simulink model "StewartDynamics"  (R2015a)
settings: Solver=ode45  StartTime=0.0  StopTime=10.0  RelTol=1e-3
settings Model: Creator=admin  LastModifiedBy=admin

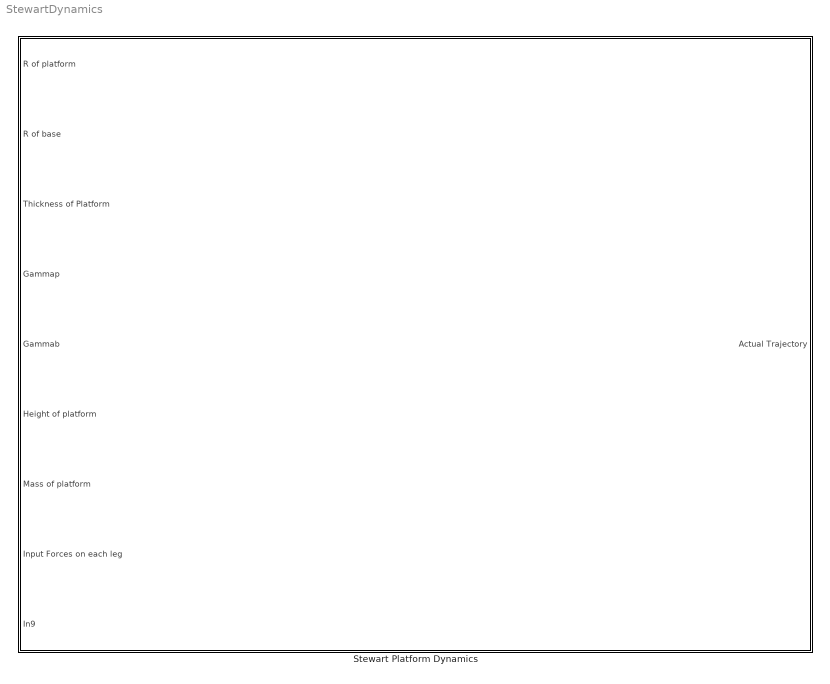
== system StewartDynamics ==
  Stewart Platform Dynamics : Subsystem

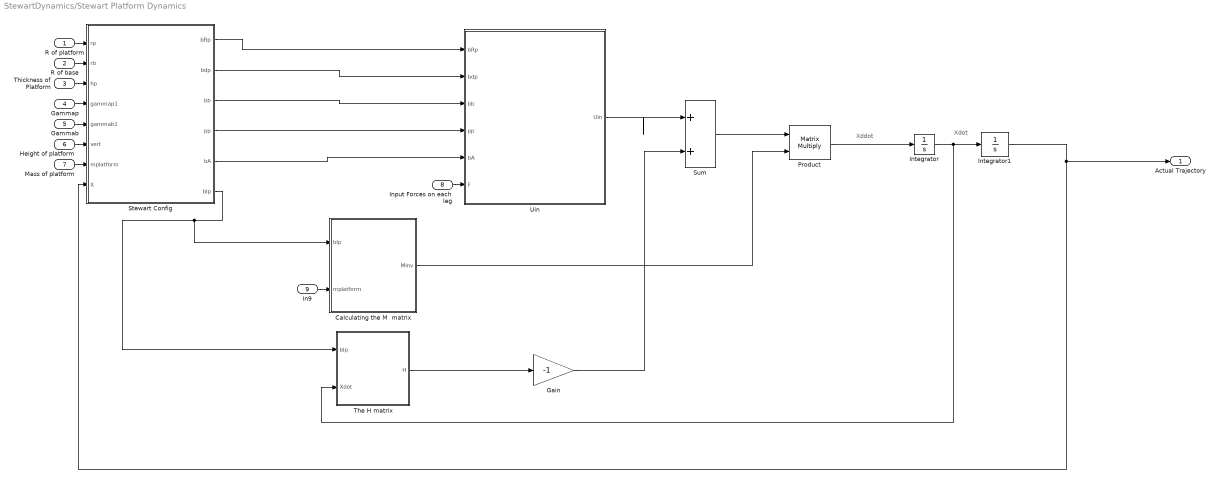
== system StewartDynamics/Stewart Platform Dynamics ==
  note: Xdot
  note: Xddot
  R of platform : Inport
  R of base : Inport  Port=2
  Thickness of Platform : Inport  Port=3
  Gammap : Inport  Port=4
  Gammab : Inport  Port=5
  "Height of platform " : Inport  Port=6
  Mass of platform : Inport  Port=7
  Input Forces on each leg : Inport  Port=8
  In9 : Inport  Port=9
  Calculating the M  matrix : MATLAB Function  TreatAsAtomicUnit=on
  Gain : Gain  Gain=-1
  Integrator : Integrator
  Integrator1 : Integrator
  Product : Product  Multiplication=Matrix(*)
  Stewart Config : MATLAB Function  TreatAsAtomicUnit=on
  Sum : Sum  Inputs=|++
  The H matrix : MATLAB Function  TreatAsAtomicUnit=on
  Uin : MATLAB Function  TreatAsAtomicUnit=on
  Actual Trajectory : Outport
  wires:
  R of platform/1 -> Stewart Config/1(rp)
  "Height of platform "/1 -> Stewart Config/6(vert)
  Input Forces on each leg/1 -> Uin/6(F)
  Gammap/1 -> Stewart Config/4(gammap1)
  Gammab/1 -> Stewart Config/5(gammab1)
  Thickness of Platform/1 -> Stewart Config/3(hp)
  In9/1 -> Calculating the M  matrix/2(mplatform)
  Mass of platform/1 -> Stewart Config/7(mplatform)
  R of base/1 -> Stewart Config/2(rb)
  Stewart Config/6(bIp) -> The H matrix/1(bIp), Calculating the M  matrix/1(bIp)
  Stewart Config/5(bA) -> Uin/5(bA)
  Stewart Config/4(pp) -> Uin/4(pp)
  Integrator1/1 -> Actual Trajectory/1, Stewart Config/8(X)
  Integrator/1 -> Integrator1/1, The H matrix/2(Xdot)
  Product/1 -> Integrator/1
  The H matrix/1(H) -> Gain/1
  Stewart Config/1(bRp) -> Uin/1(bRp)
  Calculating the M  matrix/1(Minv) -> Product/2
  Sum/1 -> Product/1
  Stewart Config/3(bb) -> Uin/3(bb)
  Uin/1(Uin) -> Sum/1
  Stewart Config/2(bdp) -> Uin/2(bdp)
  Gain/1 -> Sum/2

== matlab function StewartDynamics/Stewart Platform Dynamics/Stewart Config ==
  data: rp input; bRp output; rb input; hp input; gammap1 input; gammab1 input; vert input; mplatform input; X input; bdp output; bb output; pp output; bA output; bIp output
function [bRp,bdp,bb,pp,bA,bIp] = fcn(rp,rb,hp,gammap1,gammab1,vert,mplatform,X)
%#codegen
gammap = [gammap1,120-gammapl, 120+gammap1, -120-gammap1,-120+gammap1,-gammap1];
gammab = [gammab1,120-gammab1, 120+gammab1, -120-gammab1,-120+gammab1,-gammab1];

 %alphap = [0 , 120, 120, -120 , -120 , 0] ;  
 %betab = [60,60,180,180,-60,-60];
 
 
 % pIp = mplatform *[((rp^2)/4) , 0, 0; 0, ((rp*2)/4), 0; 0, 0, (rp^2)/2] ;
    pp=zeros(3,6);
    pp(1,: ) = rp*cos(gammap*pi/180);
    pp(2,: ) = rp*sin(gammap*pi/180) ;
    pp(3,: ) = [hp/2,hp/2,hp/2,hp/2,hp/2,hp/2 ] ;        %hp is the thickness of the platform
    bb=zeros(3,6);
    bb(1,: ) = rb*cos(gammab*pi/180);
    bb(2,: ) = rb*sin(gammab*pi/180);
    bb(3,: ) = [0 , 0, 0, 0 , 0, 0] ;
    
     bdp = [X(1,a),X(2,a),X(3,a)+vert]' ;                        %Position of platform frame wrt base
    bDp = [bdp,bdp,bdp,bdp,bdp,bdp] ;                           %This is same for all 6 actuators
   
      psi=X(4,a);
    the=X(5,a);
    phi=X(6,a);
    
   
    spsi = sin(psi);
    cpsi = cos(psi);
    sthe = sin(the);
    cthe = cos(the);
    sphi = sin(phi);
    cphi = cos(phi);
    
    
    pIp = mplatform *[((0.15^2)/4) , 0, 0; 0, ((0.15*2)/4), 0; 0, 0, (0.15^2)/2] ;
    bRp=zeros(3,3);
    bRp(1,1 ) = cphi * cthe ;
    bRp(1,2 ) = -sphi*cpsi + cphi * sthe * spsi ;
    bRp(1,3 ) = sphi * spsi + cphi * sthe * cpsi ;
    bRp(2,1 ) = sphi * cthe ;
    bRp(2,2 ) = cphi * cpsi + sphi * sthe * spsi ;
    bRp(2,3 ) = -cphi * spsi + sphi * sthe * cpsi ;
    bRp(3,1 ) = -sthe ;
    bRp(3,2 ) = cthe * spsi ;
    bRp(3,3 ) = cthe * cpsi ;
    
     bA = bRp*pp + bDp - bb ;                                    %Actuator vector
    
     bIp=bRp*pIp*bRp';                                           %Inertia tensor varying due to orientation of platform wrt base

== matlab function StewartDynamics/Stewart Platform Dynamics/Uin ==
  data: bRp input; bdp input; bb input; Uin output; pp input; bA input; F input
function Uin = fcn(bRp,bdp,bb,pp,bA,F)
%#codegen

    G=[0,0,-g]';
    Fvec=zeros(3,6);
    %We are going to add g in vector form to the input force
   
    for j=1:6
       Fvec(:,j)=F(j,a)*bA(:,j);
    end
    
    
   U=zeros(6,1);                                              %Combined effect of gravity and force on actuators
     for j=1:6
       U(j,1)= F(j,a)+dot(Fvec(:,j),G);
     end
     
    Jt=zeros(6,6);
   
      for i=1:6
      Jt(:,i ) = [ ( bRp*pp(:,i) + bdp - bb(:,i) ); cross( bRp*pp(:,i),bdp-bb(:,i) ) ] / norm(bA(:,i)) ;
  
      end
    
     Uin=Jt*U;                                                %Input u in state space form

== matlab function StewartDynamics/Stewart Platform Dynamics/Calculating the M  matrix ==
  data: bIp input; mplatform input; Minv output
function Minv = fcn(bIp,mplatform)
%#codegen

m=mplatform*(eye(3));

z=zeros(3,3);

M=[m,z;z,bIp];
Minv=inv(M);

== matlab function StewartDynamics/Stewart Platform Dynamics/The H matrix ==
  data: bIp input; H output; Xdot input
function H = fcn(bIp,Xdot)
%#codegen
bWp = [Xdot(4,1) ; Xdot(5,1) ; Xdot(6,1)] ;

bWpskew=[ 0 , -1*bWp(3,1) , bWp(2,1) ; 
         bWp(3,1) , 0 , -1*bWp(1,1)  ;
         -1*bWp(2,1), bWp(1,1), 0 ];
     
     h= bWpskew*bIp;                             %WxI
    H=[z,z;z,h];
